simulink model "przestrzen_stanu_2"  (R2014b)
settings: Solver=FixedStepDiscrete  StartTime=0.0  StopTime=10.0  RelTol=1e-3
values from neighbouring files (symbols this model uses):
  x0 = [ 10 1 10 ]    [zad_4.m]
undefined symbols (not defined in the file or in its folder): A2, B2, Tp
settings Model: Creator=Konrad  LastModifiedBy=Konrad

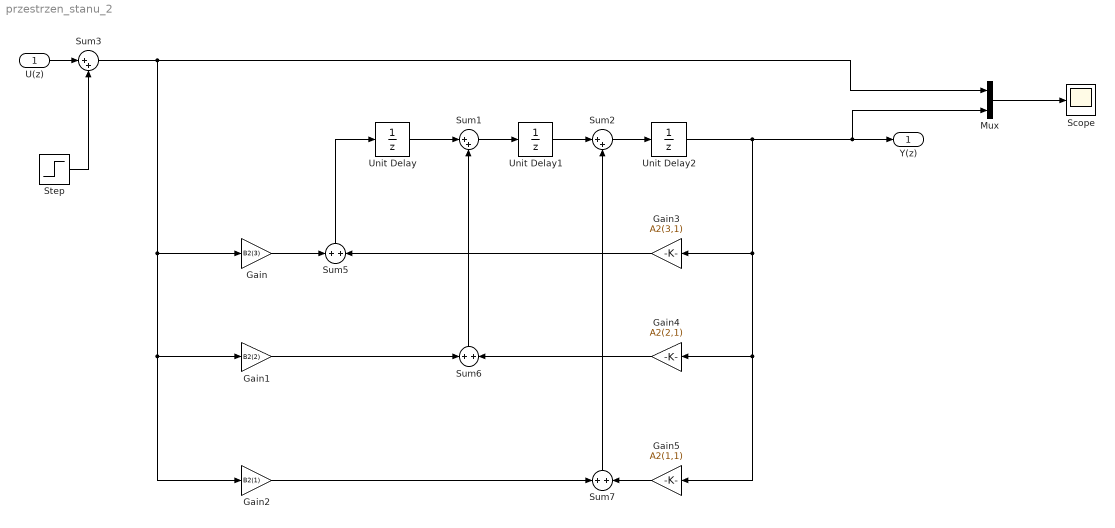
== system przestrzen_stanu_2 ==
  U(z) : Inport
  Gain : Gain  Gain=B2(3)
  Gain1 : Gain  Gain=B2(2)
  Gain2 : Gain  Gain=B2(1)
  Gain3 : Gain  Gain=A2(3,1)
  Gain4 : Gain  Gain=A2(2,1)
  Gain5 : Gain  Gain=A2(1,1)
  Mux : Mux  Inputs=2
  Scope : Scope
  Step : Step  SampleTime=0
  Sum1 : Sum  Inputs=|++
  Sum2 : Sum  Inputs=|++
  Sum3 : Sum  Inputs=|++
  Sum5 : Sum  Inputs=+|+
  Sum6 : Sum  Inputs=+|+
  Sum7 : Sum  Inputs=+|+
  Unit Delay : UnitDelay  InitialCondition=x0(3)  SampleTime=Tp
  Unit Delay1 : UnitDelay  InitialCondition=x0(2)  SampleTime=Tp
  Unit Delay2 : UnitDelay  InitialCondition=x0(1)  SampleTime=Tp
  Y(z) : Outport
  wires:
  Sum1/1 -> Unit Delay1/1
  Unit Delay1/1 -> Sum2/1
  Sum2/1 -> Unit Delay2/1
  Unit Delay/1 -> Sum1/1
  Gain/1 -> Sum5/1
  Unit Delay2/1 -> Mux/2, Y(z)/1, Gain3/1, Gain4/1, Gain5/1
  Gain3/1 -> Sum5/2
  Gain4/1 -> Sum6/2
  Gain5/1 -> Sum7/2
  Gain1/1 -> Sum6/1
  Gain2/1 -> Sum7/1
  Sum6/1 -> Sum1/2
  Sum7/1 -> Sum2/2
  Sum3/1 -> Mux/1, Gain/1, Gain1/1, Gain2/1
  Sum5/1 -> Unit Delay/1
  Mux/1 -> Scope/1
  Step/1 -> Sum3/2
  U(z)/1 -> Sum3/1
